simulink model "TRN"  (R2022a)
settings: Solver=FixedStepAuto  StartTime=0.0  StopTime=300  FixedStep=0.04  RelTol=1e-3
PreLoadFcn:
  | load('BusStructureTRNsensor.mat');
  | addpath('C:/MAP');
InitFcn:
  | %load TRNDataBusPILS.mat
  | %addpath(genpath(cd))
  | 
  | load('TPF_WHOLESIM_INPUT_SCENARIOS_AGCAS_N35_10E127_70.mat');
  | 
  | % Add DataBus Path
  | addpath(',,/');
  | addpath('../MAP/');
  | addpath('../MAP/MAP_DB');
  | addpath('../MAP/DVOF');
  | addpath(genpath(cd));
  | load('BusStructureTRN.mat');
undefined symbols (not defined in the file or in its folder): Altitude_INS, INSDataNotValid, Latitude_INS, Longitude_INS, TRN, TRNlib
libraries: simulink_extras x26, aerolibconvert2 x14, sharedtransform x3, dspstat3 x2
(part 2 of 3)

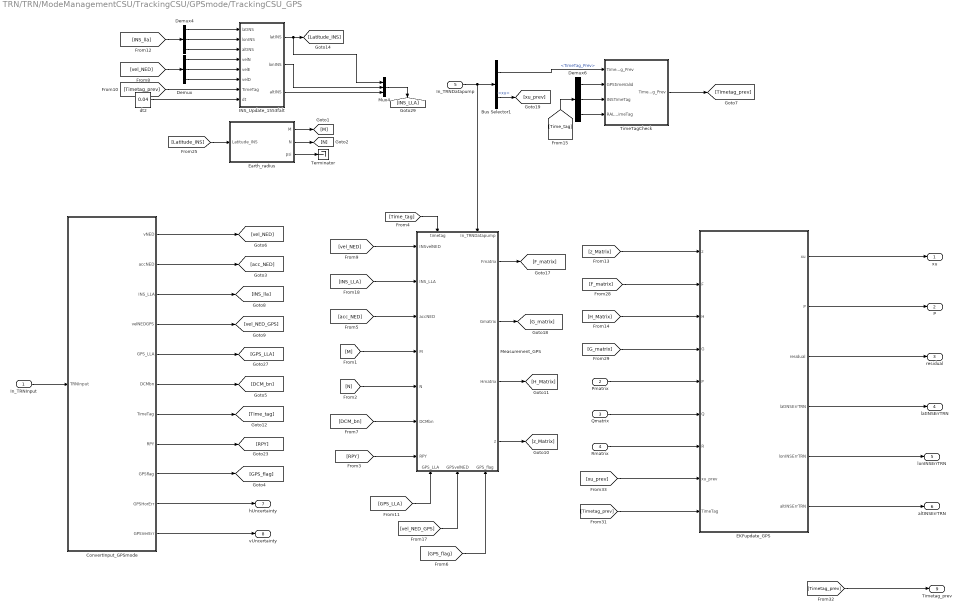
== system TRN/TRN/ModeManagementCSU/TrackingCSU/GPSmode/TrackingCSU_GPS ==
  In_TRNInput : Inport  OutDataTypeStr=Bus: TRNInput
  Pmatrix : Inport  Port=2
  Qmatrix : Inport  Port=3
  Rmatrix : Inport  Port=4
  In_TRNDatapump : Inport  Port=5  OutDataTypeStr=Bus: TRNDatapump  PortDimensions=1
  Bus Selector1 : BusSelector  OutputSignals=TimeTag_Prev,xu
  ConvertInput_GPSmode : Subsystem  TreatAsAtomicUnit=on
  Demux : Demux  Outputs=3
  Demux4 : Demux  Outputs=3
  Demux6 : Demux  Outputs=3
  EKFupdate_GPS : Subsystem
  Earth_radius : MATLAB Function  TreatAsAtomicUnit=on
  INS_Update_1553falt : MATLAB Function  TreatAsAtomicUnit=on
  Measurement_GPS : Subsystem
      settings: PortSchema="{\"entries\":[{\"content\":{\"sides\":[{\"content\":{\"connectorIds\":[\"In1\",\"In2\",\"In3\",\"In4\",\"In5\",\"In6\",\"In7\"]},\"type\":\"ConnectorPlacement.EquallySpacedRectSide\",\"uuid\":\"284c5e42-61c1-4616-966e-143f60f46571\"},{\"content\":{\"connectorIds\":[\"Out1\",\"Out2\",\"Out3\",\"Out4\"],\"side\":\"RIGHT\"},\"type\":\"ConnectorPlacement.EquallySpacedRectSide\",\"uuid\":\"be5b0b09-4e69-4cdf-8a94-a8639994cbf9\"},{\"content\":{\"connectorIds\":[\"In8\",\"In9\"],\"side\":\"TOP\"},\"type\":\"ConnectorPlacement.EquallySpacedRectSide\",\"uuid\":\"f7fbee8b-afe7-4fec-8c40-a5bd5e14374e\"},{\"content\":{\"connectorIds\":[\"In10\",\"In11\",\"In12\"],\"side\":\"BOTTOM\"},\"type\":\"ConnectorPlacement.EquallySpacedRectSide\",\"uuid\":\"9a503e43-aaca-441a-ab76-b52386228bc3\"}]},\"type\":\"ConnectorPlacement.EquallySpacedConnector\",\"uuid\":\"1b32203e-baad-4c49-8c24-20b6a9ecb4b9\"}],\"packageUris\":[\"http://schema.mathworks.com/mf0/Connector/R2020b\"],\"version\":\"1.0\"}"
  Mux4 : Mux  Inputs=3
  Terminator : Terminator
  TimeTagCheck : MATLAB Function  TreatAsAtomicUnit=on
  dt2 : Constant  Value=0.04  OutDataTypeStr=double
  xu : Outport
  P : Outport  Port=2
  residual : Outport  Port=3
  latINSErrTRN : Outport  Port=4
  lonINSErrTRN : Outport  Port=5
  altINSErrTRN : Outport  Port=6
  hUncertainty : Outport  Port=7
  vUncertainty : Outport  Port=8
  Timetag_prev : Outport  Port=9
  wires:
  Mux4/1 -> [INS_LLA]
  Demux/3 -> INS_Update_1553falt/6(velD)
  Demux/1 -> INS_Update_1553falt/4(velN)
  Demux/2 -> INS_Update_1553falt/5(velE)
  dt2/1 -> INS_Update_1553falt/8(dt)
  Bus Selector1/1 -> TimeTagCheck/1("TimeTag_Prev ")  "<TimeTag_Prev>"
  In_TRNDatapump/1 -> Bus Selector1/1, Measurement_GPS/9(In_TRNDatapump)
  INS_Update_1553falt/3(altINS) -> Mux4/3
  In_TRNInput/1 -> ConvertInput_GPSmode/1(TRNInput)
  INS_Update_1553falt/1(latINS) -> [Latitude_INS], Mux4/1
  INS_Update_1553falt/2(lonINS) -> Mux4/2
  ConvertInput_GPSmode/2(accNED) -> [acc_NED]
  ConvertInput_GPSmode/6(DCMbn) -> [DCM_bn]
  ConvertInput_GPSmode/1(vNED) -> [vel_NED]
  [vel_NED] -> Demux/1
  [Timetag_prev] -> INS_Update_1553falt/7(TimeTag)
  [INS_lla] -> Demux4/1
  Demux4/2 -> INS_Update_1553falt/2("lonINS ")
  Demux4/1 -> INS_Update_1553falt/1("latINS ")
  Demux4/3 -> INS_Update_1553falt/3("altINS ")
  ConvertInput_GPSmode/4(velNEDGPS) -> [vel_NED_GPS]
  [Time_tag] -> Demux6/1
  Demux6/1 -> TimeTagCheck/2(GPStimeValid)
  Demux6/2 -> TimeTagCheck/3(INSTimeTag)
  Demux6/3 -> TimeTagCheck/4(RALTTimeTag)
  [Timetag_prev] -> Timetag_prev/1
  Bus Selector1/2 -> [xu_prev]  "<xu>"
  Measurement_GPS/1(Fmatrix) -> [F_matrix]
  Measurement_GPS/2(Gmatrix) -> [G_matrix]
  Measurement_GPS/3(Hmatrix) -> [H_Matrix]
  Measurement_GPS/4(z) -> [z_Matrix]
  [z_Matrix] -> EKFupdate_GPS/1(z)
  [F_matrix] -> EKFupdate_GPS/2(F)
  [H_Matrix] -> EKFupdate_GPS/3(H)
  [G_matrix] -> EKFupdate_GPS/4(G)
  Pmatrix/1 -> EKFupdate_GPS/5("P ")
  Qmatrix/1 -> EKFupdate_GPS/6(Q)
  [xu_prev] -> EKFupdate_GPS/8(xu_prev)
  [Timetag_prev] -> EKFupdate_GPS/9(TimeTag)
  EKFupdate_GPS/1(xu) -> xu/1
  EKFupdate_GPS/2(P) -> P/1
  EKFupdate_GPS/3(residual) -> residual/1
  EKFupdate_GPS/4(latINSErrTRN) -> latINSErrTRN/1
  EKFupdate_GPS/5(lonINSErrTRN) -> lonINSErrTRN/1
  EKFupdate_GPS/6(altINSErrTRN) -> altINSErrTRN/1
  [vel_NED] -> Measurement_GPS/1(INSvelNED)
  [INS_LLA] -> Measurement_GPS/2(INS_LLA)
  [acc_NED] -> Measurement_GPS/3(accNED)
  [M] -> Measurement_GPS/4(M)
  [N] -> Measurement_GPS/5(N)
  [Latitude_INS] -> Earth_radius/1(Latitude_INS)
  Earth_radius/1(M) -> [M]
  Earth_radius/2(N) -> [N]
  ConvertInput_GPSmode/5(GPS_LLA) -> [GPS_LLA]
  [DCM_bn] -> Measurement_GPS/6(DCMbn)
  ConvertInput_GPSmode/8(RPY) -> [RPY]
  [RPY] -> Measurement_GPS/7(RPY)
  TimeTagCheck/1(TimeTag_Prev) -> [Timetag_prev]
  [GPS_LLA] -> Measurement_GPS/10(GPS_LLA)
  [vel_NED_GPS] -> Measurement_GPS/11(GPSvelNED)
  Rmatrix/1 -> EKFupdate_GPS/7(R)
  [Time_tag] -> Measurement_GPS/8(timetag)
  ConvertInput_GPSmode/9(GPSflag) -> [GPS_flag]
  [GPS_flag] -> Measurement_GPS/12(GPS_flag)
  ConvertInput_GPSmode/10(GPSHorErr) -> hUncertainty/1
  ConvertInput_GPSmode/11(GPSVerErr) -> vUncertainty/1
  ConvertInput_GPSmode/7(TimeTag) -> [Time_tag]
  ConvertInput_GPSmode/3(INS_LLA) -> [INS_lla]
  Earth_radius/3(psi) -> Terminator/1

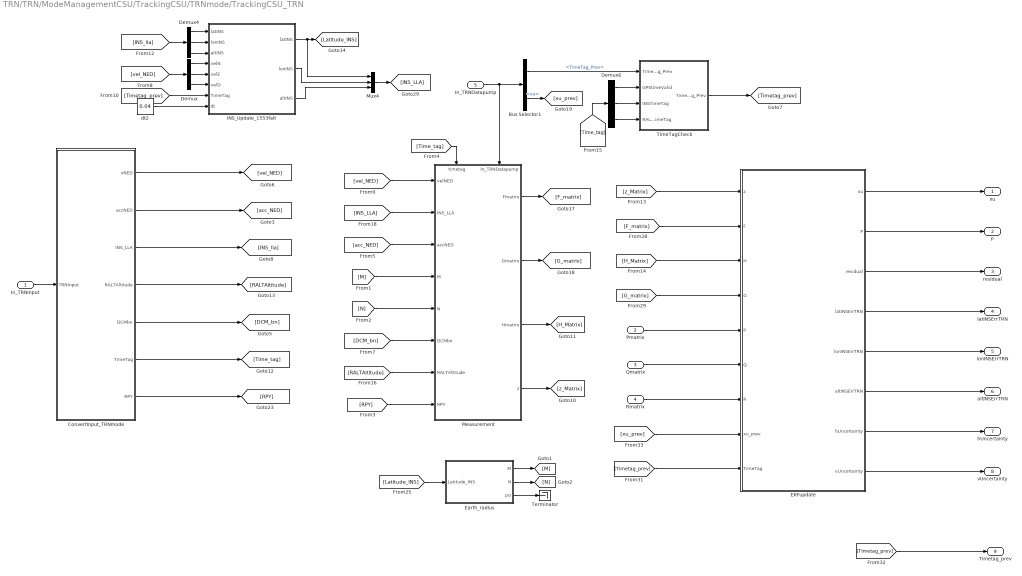
== system TRN/TRN/ModeManagementCSU/TrackingCSU/TRNmode/TrackingCSU_TRN ==
  In_TRNInput : Inport  OutDataTypeStr=Bus: TRNInput
  Pmatrix : Inport  Port=2
  Qmatrix : Inport  Port=3
  Rmatrix : Inport  Port=4
  In_TRNDatapump : Inport  Port=5  OutDataTypeStr=Bus: TRNDatapump  PortDimensions=1
  Bus Selector1 : BusSelector  OutputSignals=TimeTag_Prev,xu
  ConvertInput_TRNmode : Subsystem  TreatAsAtomicUnit=on
  Demux : Demux  Outputs=3
  Demux4 : Demux  Outputs=3
  Demux6 : Demux  Outputs=3
  EKFupdate : Subsystem
  Earth_radius : MATLAB Function  TreatAsAtomicUnit=on
  INS_Update_1553falt : MATLAB Function  TreatAsAtomicUnit=on
  Measurement : Subsystem
      settings: PortSchema="{\"entries\":[{\"content\":{\"sides\":[{\"content\":{\"connectorIds\":[\"In1\",\"In2\",\"In3\",\"In4\",\"In5\",\"In6\",\"In7\",\"In8\"]},\"type\":\"ConnectorPlacement.EquallySpacedRectSide\",\"uuid\":\"284c5e42-61c1-4616-966e-143f60f46571\"},{\"content\":{\"connectorIds\":[\"Out1\",\"Out2\",\"Out3\",\"Out4\"],\"side\":\"RIGHT\"},\"type\":\"ConnectorPlacement.EquallySpacedRectSide\",\"uuid\":\"be5b0b09-4e69-4cdf-8a94-a8639994cbf9\"},{\"content\":{\"connectorIds\":[\"In9\",\"In10\"],\"side\":\"TOP\"},\"type\":\"ConnectorPlacement.EquallySpacedRectSide\",\"uuid\":\"f7fbee8b-afe7-4fec-8c40-a5bd5e14374e\"}]},\"type\":\"ConnectorPlacement.EquallySpacedConnector\",\"uuid\":\"1b32203e-baad-4c49-8c24-20b6a9ecb4b9\"}],\"packageUris\":[\"http://schema.mathworks.com/mf0/Connector/R2020b\"],\"version\":\"1.0\"}"
  Mux4 : Mux  Inputs=3
  Terminator : Terminator
  TimeTagCheck : MATLAB Function  TreatAsAtomicUnit=on
  dt2 : Constant  Value=0.04  OutDataTypeStr=double
  xu : Outport
  P : Outport  Port=2
  residual : Outport  Port=3
  latINSErrTRN : Outport  Port=4
  lonINSErrTRN : Outport  Port=5
  altINSErrTRN : Outport  Port=6
  hUncertainty : Outport  Port=7
  vUncertainty : Outport  Port=8
  Timetag_prev : Outport  Port=9
  wires:
  TimeTagCheck/1(TimeTag_Prev) -> [Timetag_prev]
  [RPY] -> Measurement/8(RPY)
  ConvertInput_TRNmode/7(RPY) -> [RPY]
  [DCM_bn] -> Measurement/6(DCMbn)
  [RALTAltitude] -> Measurement/7(RALTAltitude)
  [N] -> Measurement/5(N)
  [M] -> Measurement/4(M)
  [acc_NED] -> Measurement/3(accNED)
  [INS_LLA] -> Measurement/2(INS_LLA)
  [vel_NED] -> Measurement/1(velNED)
  EKFupdate/7(hUncertainty) -> hUncertainty/1
  EKFupdate/6(altINSErrTRN) -> altINSErrTRN/1
  EKFupdate/5(lonINSErrTRN) -> lonINSErrTRN/1
  EKFupdate/4(latINSErrTRN) -> latINSErrTRN/1
  EKFupdate/8(vUncertainty) -> vUncertainty/1
  EKFupdate/3(residual) -> residual/1
  EKFupdate/2(P) -> P/1
  EKFupdate/1(xu) -> xu/1
  [Timetag_prev] -> EKFupdate/9(TimeTag)
  [xu_prev] -> EKFupdate/8(xu_prev)
  Rmatrix/1 -> EKFupdate/7(R)
  Qmatrix/1 -> EKFupdate/6(Q)
  Pmatrix/1 -> EKFupdate/5("P ")
  [G_matrix] -> EKFupdate/4(G)
  [H_Matrix] -> EKFupdate/3(H)
  [F_matrix] -> EKFupdate/2(F)
  [z_Matrix] -> EKFupdate/1(z)
  Measurement/4(z) -> [z_Matrix]
  Measurement/3(Hmatrix) -> [H_Matrix]
  Measurement/2(Gmatrix) -> [G_matrix]
  Measurement/1(Fmatrix) -> [F_matrix]
  Bus Selector1/2 -> [xu_prev]  "<xu>"
  [Timetag_prev] -> Timetag_prev/1
  ConvertInput_TRNmode/4(RALTAltitude) -> [RALTAltitude]
  Demux6/3 -> TimeTagCheck/4(RALTTimeTag)
  Demux6/2 -> TimeTagCheck/3(INSTimeTag)
  Demux6/1 -> TimeTagCheck/2(GPStimeValid)
  [Time_tag] -> Demux6/1
  Demux4/3 -> INS_Update_1553falt/3("altINS ")
  Demux4/1 -> INS_Update_1553falt/1("latINS ")
  Demux4/2 -> INS_Update_1553falt/2("lonINS ")
  [INS_lla] -> Demux4/1
  [Timetag_prev] -> INS_Update_1553falt/7(TimeTag)
  [vel_NED] -> Demux/1
  ConvertInput_TRNmode/1(vNED) -> [vel_NED]
  ConvertInput_TRNmode/5(DCMbn) -> [DCM_bn]
  ConvertInput_TRNmode/2(accNED) -> [acc_NED]
  INS_Update_1553falt/2(lonINS) -> Mux4/2
  INS_Update_1553falt/1(latINS) -> Mux4/1, [Latitude_INS]
  In_TRNInput/1 -> ConvertInput_TRNmode/1(TRNInput)
  INS_Update_1553falt/3(altINS) -> Mux4/3
  In_TRNDatapump/1 -> Measurement/10(In_TRNDatapump), Bus Selector1/1
  Bus Selector1/1 -> TimeTagCheck/1("TimeTag_Prev ")  "<TimeTag_Prev>"
  dt2/1 -> INS_Update_1553falt/8(dt)
  Demux/2 -> INS_Update_1553falt/5(velE)
  Demux/1 -> INS_Update_1553falt/4(velN)
  Demux/3 -> INS_Update_1553falt/6(velD)
  Mux4/1 -> [INS_LLA]
  [Time_tag] -> Measurement/9(timetag)
  ConvertInput_TRNmode/6(TimeTag) -> [Time_tag]
  ConvertInput_TRNmode/3(INS_LLA) -> [INS_lla]
  Earth_radius/2(N) -> [N]
  Earth_radius/1(M) -> [M]
  [Latitude_INS] -> Earth_radius/1(Latitude_INS)
  Earth_radius/3(psi) -> Terminator/1

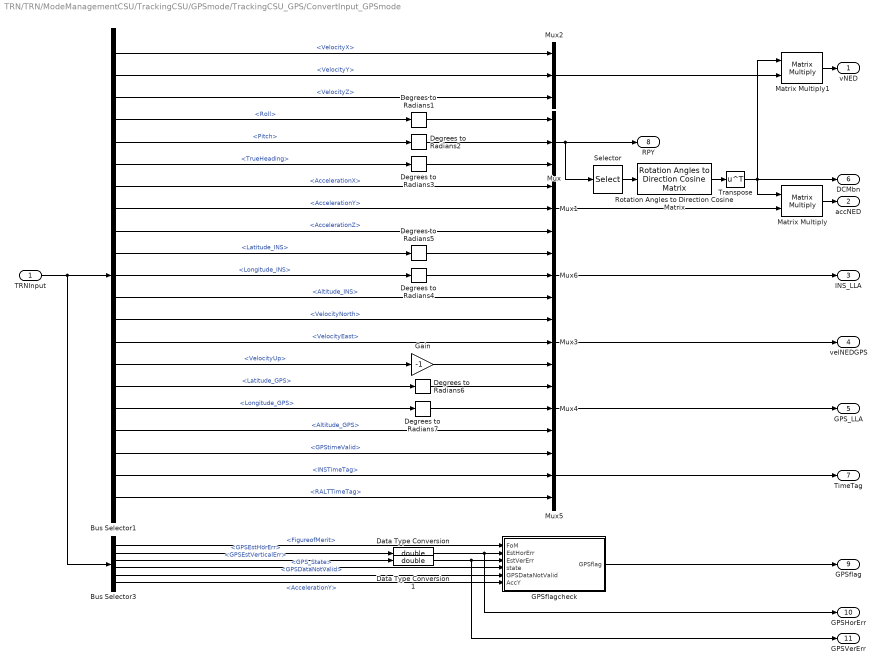
== system TRN/TRN/ModeManagementCSU/TrackingCSU/GPSmode/TrackingCSU_GPS/ConvertInput_GPSmode ==
  TRNInput : Inport
  Bus Selector1 : BusSelector  OutputSignals=VelocityX,VelocityY,VelocityZ,Roll,Pitch,TrueHeading,AccelerationX,AccelerationY,AccelerationZ,Latitude_INS,Longitude_INS,Altitude_INS,VelocityNorth,VelocityEast,VelocityUp,Latitude_GPS,Longitude_GPS,Altitude_GPS,GPStimeValid,INSTimeTag,RALTTimeTag
  Bus Selector3 : BusSelector  OutputSignals=FigureofMerit,GPSEstHorErr,GPSEstVerticalErr,GPS_State,GPSDataNotValid,AccelerationY
  Data Type Conversion : DataTypeConversion  OutDataTypeStr=double  SaturateOnIntegerOverflow=off  RndMeth=Floor
  Data Type Conversion1 : DataTypeConversion  OutDataTypeStr=double  SaturateOnIntegerOverflow=off  RndMeth=Floor
  Degrees to Radians{1..7} (7 alike) : simulink_extras/Transformations/Degrees to Radians
  GPSflagcheck : MATLAB Function  TreatAsAtomicUnit=on
  Gain : Gain  Gain=-1
  Matrix Multiply : Product  Multiplication=Matrix(*)
  Matrix Multiply1 : Product  Multiplication=Matrix(*)
  Mux{,1..6} (7 alike) : Mux  Inputs=3
  Rotation Angles to Direction Cosine Matrix : sharedtransform/Rotation Angles to Direction Cosine Matrix  rotationOrder=ZYX  aMode=aMode
      settings: SourceProductBaseCode=AE,PW,DR,MT,VE
  Selector : Selector  InputPortWidth=3  IndexOptions=Index vector (dialog)  Indices=[3 2 1]  OutputSizes=1
  Transpose : Math  Operator=transpose  SignedPower=on
  vNED : Outport  VectorParamsAs1DForOutWhenUnconnected=off
  accNED : Outport  Port=2  VectorParamsAs1DForOutWhenUnconnected=off
  INS_LLA : Outport  Port=3  VectorParamsAs1DForOutWhenUnconnected=off
  velNEDGPS : Outport  Port=4  VectorParamsAs1DForOutWhenUnconnected=off
  GPS_LLA : Outport  Port=5
  DCMbn : Outport  Port=6  VectorParamsAs1DForOutWhenUnconnected=off
  TimeTag : Outport  Port=7  VectorParamsAs1DForOutWhenUnconnected=off
  RPY : Outport  Port=8  VectorParamsAs1DForOutWhenUnconnected=off
  GPSflag : Outport  Port=9  VectorParamsAs1DForOutWhenUnconnected=off
  GPSHorErr : Outport  Port=10  VectorParamsAs1DForOutWhenUnconnected=off
  GPSVerErr : Outport  Port=11  VectorParamsAs1DForOutWhenUnconnected=off
  wires:
  Bus Selector1/18 -> Mux4/3  "<Altitude_GPS>"
  Bus Selector1/17 -> Degrees to Radians7/1  "<Longitude_GPS>"
  Degrees to Radians7/1 -> Mux4/2
  Bus Selector1/21 -> Mux5/3  "<RALTTimeTag>"
  Bus Selector1/20 -> Mux5/2  "<INSTimeTag>"
  Bus Selector1/19 -> Mux5/1  "<GPStimeValid>"
  Gain/1 -> Mux3/3
  Bus Selector1/15 -> Gain/1  "<VelocityUp>"
  Bus Selector1/14 -> Mux3/2  "<VelocityEast>"
  Bus Selector1/13 -> Mux3/1  "<VelocityNorth>"
  Bus Selector1/3 -> Mux2/3  "<VelocityZ>"
  Bus Selector1/1 -> Mux2/1  "<VelocityX>"
  Bus Selector1/4 -> Degrees to Radians1/1  "<Roll>"
  Bus Selector1/2 -> Mux2/2  "<VelocityY>"
  TRNInput/1 -> Bus Selector3/1, Bus Selector1/1
  Bus Selector1/6 -> Degrees to Radians3/1  "<TrueHeading>"
  Degrees to Radians2/1 -> Mux/2
  Degrees to Radians3/1 -> Mux/3
  Mux/1 -> Selector/1, RPY/1
  Bus Selector1/7 -> Mux1/1  "<AccelerationX>"
  Bus Selector1/5 -> Degrees to Radians2/1  "<Pitch>"
  Degrees to Radians1/1 -> Mux/1
  Bus Selector1/9 -> Mux1/3  "<AccelerationZ>"
  Bus Selector1/8 -> Mux1/2  "<AccelerationY>"
  Matrix Multiply1/1 -> vNED/1
  Matrix Multiply/1 -> accNED/1
  Mux1/1 -> Matrix Multiply/2
  Bus Selector1/10 -> Degrees to Radians5/1  "<Latitude_INS>"
  Transpose/1 -> Matrix Multiply/1, DCMbn/1, Matrix Multiply1/1
  Mux2/1 -> Matrix Multiply1/2
  Rotation Angles to Direction Cosine Matrix/1 -> Transpose/1
  Bus Selector1/11 -> Degrees to Radians4/1  "<Longitude_INS>"
  Degrees to Radians6/1 -> Mux4/1
  Bus Selector1/16 -> Degrees to Radians6/1  "<Latitude_GPS>"
  Selector/1 -> Rotation Angles to Direction Cosine Matrix/1
  Bus Selector3/2 -> Data Type Conversion/1  "<GPSEstHorErr>"
  Bus Selector3/1 -> GPSflagcheck/1(FoM)  "<FigureofMerit>"
  Bus Selector3/5 -> GPSflagcheck/5(GPSDataNotValid)  "<GPSDataNotValid>"
  Bus Selector3/3 -> Data Type Conversion1/1  "<GPSEstVerticalErr>"
  Bus Selector3/4 -> GPSflagcheck/4(state)  "<GPS_State>"
  Mux4/1 -> GPS_LLA/1
  Mux3/1 -> velNEDGPS/1
  GPSflagcheck/1(GPSflag) -> GPSflag/1
  Bus Selector3/6 -> GPSflagcheck/6(AccY)  "<AccelerationY>"
  Data Type Conversion/1 -> GPSHorErr/1, GPSflagcheck/2(EstHorErr)
  Data Type Conversion1/1 -> GPSVerErr/1, GPSflagcheck/3(EstVerErr)
  Mux5/1 -> TimeTag/1
  Degrees to Radians5/1 -> Mux6/1
  Degrees to Radians4/1 -> Mux6/2
  Bus Selector1/12 -> Mux6/3  "<Altitude_INS>"
  Mux6/1 -> INS_LLA/1

== system TRN/TRN/ModeManagementCSU/TrackingCSU/GPSmode/TrackingCSU_GPS/EKFupdate_GPS ==
  z : Inport
  F : Inport  Port=2
  H : Inport  Port=3
  G : Inport  Port=4
  "P " : Inport  Port=5
  Q : Inport  Port=6
  R : Inport  Port=7
  xu_prev : Inport  Port=8
  TimeTag : Inport  Port=9
  EKFUpdate_GPS : MATLAB Function  TreatAsAtomicUnit=on
  dt3 : Constant  Value=0.04  OutDataTypeStr=double
  xu : Outport
  P : Outport  Port=2
  residual : Outport  Port=3
  latINSErrTRN : Outport  Port=4
  lonINSErrTRN : Outport  Port=5
  altINSErrTRN : Outport  Port=6
  wires:
  R/1 -> EKFUpdate_GPS/7(R)
  H/1 -> EKFUpdate_GPS/3(H)
  "P "/1 -> EKFUpdate_GPS/5("P ")
  EKFUpdate_GPS/3(residual) -> residual/1
  TimeTag/1 -> EKFUpdate_GPS/10(TimeTag)
  F/1 -> EKFUpdate_GPS/2(F)
  xu_prev/1 -> EKFUpdate_GPS/9(xu_prev)
  G/1 -> EKFUpdate_GPS/4(G)
  EKFUpdate_GPS/1(xu) -> xu/1
  EKFUpdate_GPS/2(P) -> P/1
  Q/1 -> EKFUpdate_GPS/6(Q)
  z/1 -> EKFUpdate_GPS/1(z)
  dt3/1 -> EKFUpdate_GPS/8(dt)
  EKFUpdate_GPS/4(latINSErrTRN) -> latINSErrTRN/1
  EKFUpdate_GPS/5(lonINSErrTRN) -> lonINSErrTRN/1
  EKFUpdate_GPS/6(altINSErrTRN) -> altINSErrTRN/1

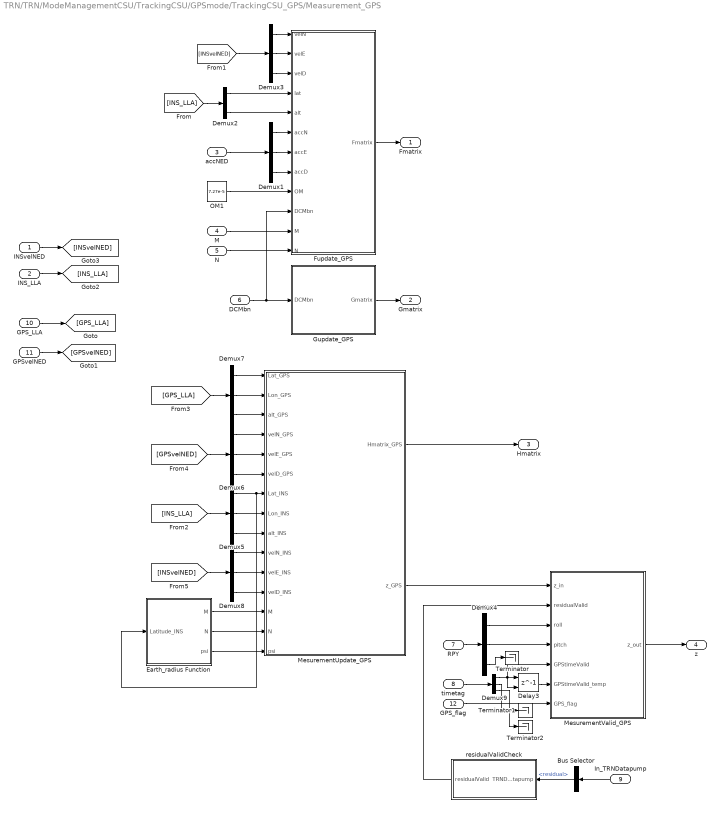
== system TRN/TRN/ModeManagementCSU/TrackingCSU/GPSmode/TrackingCSU_GPS/Measurement_GPS ==
  INSvelNED : Inport
  INS_LLA : Inport  Port=2
  accNED : Inport  Port=3
  M : Inport  Port=4
  N : Inport  Port=5
  DCMbn : Inport  Port=6
  RPY : Inport  Port=7
  timetag : Inport  Port=8
  In_TRNDatapump : Inport  Port=9
  GPS_LLA : Inport  Port=10
  GPSvelNED : Inport  Port=11
  GPS_flag : Inport  Port=12
  Bus Selector : BusSelector  OutputSignals=residual
  Delay3 : Delay  DelayLength=1  InitialConditionSource=Input port
      settings: InputPortMap=u0,p4
  Demux{1..9} (9 alike) : Demux  Outputs=3
  Earth_radius Function : MATLAB Function  TreatAsAtomicUnit=on
  Fupdate_GPS : MATLAB Function  TreatAsAtomicUnit=on
  Gupdate_GPS : MATLAB Function  TreatAsAtomicUnit=on
  MesurementUpdate_GPS : MATLAB Function  TreatAsAtomicUnit=on
  MesurementValid_GPS : MATLAB Function  TreatAsAtomicUnit=on
  OM1 : Constant  Value=7.27e-5
  Terminator : Terminator
  Terminator1 : Terminator
  Terminator2 : Terminator
  residualValidCheck : Subsystem
  Fmatrix : Outport
  Gmatrix : Outport  Port=2
  Hmatrix : Outport  Port=3
  z : Outport  Port=4
  wires:
  Demux1/3 -> Fupdate_GPS/8(accD)
  OM1/1 -> Fupdate_GPS/9(OM)
  Demux3/1 -> Fupdate_GPS/1(velN)
  Demux1/2 -> Fupdate_GPS/7(accE)
  Demux3/3 -> Fupdate_GPS/3(velD)
  Demux3/2 -> Fupdate_GPS/2(velE)
  Demux1/1 -> Fupdate_GPS/6(accN)
  Fupdate_GPS/1(Fmatrix) -> Fmatrix/1
  DCMbn/1 -> Gupdate_GPS/1(DCMbn), Fupdate_GPS/10(DCMbn)
  N/1 -> Fupdate_GPS/12(N)
  accNED/1 -> Demux1/1
  M/1 -> Fupdate_GPS/11(M)
  Demux2/1 -> Fupdate_GPS/4(lat)
  Demux2/3 -> Fupdate_GPS/5(alt)
  RPY/1 -> Demux4/1
  In_TRNDatapump/1 -> Bus Selector/1
  Bus Selector/1 -> residualValidCheck/1(TRNDatapump)  "<residual>"
  Demux5/1 -> Earth_radius Function/1(Latitude_INS), MesurementUpdate_GPS/7(Lat_INS)
  Demux5/2 -> MesurementUpdate_GPS/8(Lon_INS)
  Demux5/3 -> MesurementUpdate_GPS/9(alt_INS)
  Demux6/1 -> MesurementUpdate_GPS/4(velN_GPS)
  Demux6/2 -> MesurementUpdate_GPS/5(velE_GPS)
  Demux6/3 -> MesurementUpdate_GPS/6(velD_GPS)
  Demux7/1 -> MesurementUpdate_GPS/1(Lat_GPS)
  Demux7/2 -> MesurementUpdate_GPS/2(Lon_GPS)
  Demux7/3 -> MesurementUpdate_GPS/3(alt_GPS)
  Demux8/1 -> MesurementUpdate_GPS/10(velN_INS)
  Demux8/2 -> MesurementUpdate_GPS/11(velE_INS)
  Demux8/3 -> MesurementUpdate_GPS/12(velD_INS)
  Earth_radius Function/1(M) -> MesurementUpdate_GPS/13(M)
  Earth_radius Function/2(N) -> MesurementUpdate_GPS/14(N)
  Earth_radius Function/3(psi) -> MesurementUpdate_GPS/15(psi)
  GPS_LLA/1 -> [GPS_LLA]
  GPSvelNED/1 -> [GPSvelNED]
  INS_LLA/1 -> [INS_LLA]
  [INS_LLA] -> Demux2/1
  INSvelNED/1 -> [INSvelNED]
  [INSvelNED] -> Demux3/1
  [INS_LLA] -> Demux5/1
  [GPS_LLA] -> Demux7/1
  [GPSvelNED] -> Demux6/1
  [INSvelNED] -> Demux8/1
  MesurementUpdate_GPS/2(z_GPS) -> MesurementValid_GPS/1(z_in)
  MesurementUpdate_GPS/1(Hmatrix_GPS) -> Hmatrix/1
  Gupdate_GPS/1(Gmatrix) -> Gmatrix/1
  MesurementValid_GPS/1(z_out) -> z/1
  timetag/1 -> Demux9/1
  Delay3/1 -> MesurementValid_GPS/6(GPStimeValid_temp)
  Demux4/1 -> MesurementValid_GPS/3(roll)
  Demux4/2 -> MesurementValid_GPS/4(pitch)
  Demux9/1 -> Delay3/2, MesurementValid_GPS/5(GPStimeValid), Delay3/1
  residualValidCheck/1(residualValid) -> MesurementValid_GPS/2(residualValid)
  GPS_flag/1 -> MesurementValid_GPS/7(GPS_flag)
  Demux4/3 -> Terminator/1
  Demux9/2 -> Terminator1/1
  Demux9/3 -> Terminator2/1

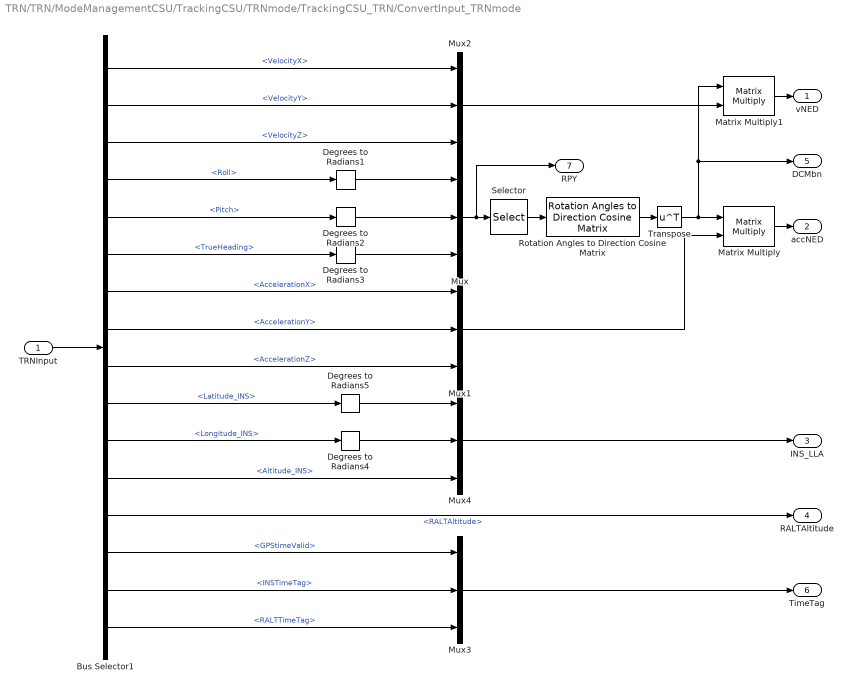
== system TRN/TRN/ModeManagementCSU/TrackingCSU/TRNmode/TrackingCSU_TRN/ConvertInput_TRNmode ==
  TRNInput : Inport
  Bus Selector1 : BusSelector  OutputSignals=VelocityX,VelocityY,VelocityZ,Roll,Pitch,TrueHeading,AccelerationX,AccelerationY,AccelerationZ,Latitude_INS,Longitude_INS,Altitude_INS,RALTAltitude,GPStimeValid,INSTimeTag,RALTTimeTag
  Degrees to Radians{1..5} (5 alike) : simulink_extras/Transformations/Degrees to Radians
  Matrix Multiply : Product  Multiplication=Matrix(*)
  Matrix Multiply1 : Product  Multiplication=Matrix(*)
  Mux{,1..4} (5 alike) : Mux  Inputs=3
  Rotation Angles to Direction Cosine Matrix : sharedtransform/Rotation Angles to Direction Cosine Matrix  rotationOrder=ZYX  aMode=aMode
      settings: SourceProductBaseCode=AE,PW,DR,MT,VE
  Selector : Selector  InputPortWidth=3  IndexOptions=Index vector (dialog)  Indices=[3 2 1]  OutputSizes=1
  Transpose : Math  Operator=transpose  SignedPower=on
  vNED : Outport  VectorParamsAs1DForOutWhenUnconnected=off
  accNED : Outport  Port=2  VectorParamsAs1DForOutWhenUnconnected=off
  INS_LLA : Outport  Port=3  VectorParamsAs1DForOutWhenUnconnected=off
  RALTAltitude : Outport  Port=4  VectorParamsAs1DForOutWhenUnconnected=off
  DCMbn : Outport  Port=5  VectorParamsAs1DForOutWhenUnconnected=off
  TimeTag : Outport  Port=6  VectorParamsAs1DForOutWhenUnconnected=off
  RPY : Outport  Port=7  VectorParamsAs1DForOutWhenUnconnected=off
  wires:
  Bus Selector1/11 -> Degrees to Radians4/1  "<Longitude_INS>"
  Rotation Angles to Direction Cosine Matrix/1 -> Transpose/1
  Mux2/1 -> Matrix Multiply1/2
  Transpose/1 -> Matrix Multiply/1, Matrix Multiply1/1, DCMbn/1
  Bus Selector1/10 -> Degrees to Radians5/1  "<Latitude_INS>"
  Mux1/1 -> Matrix Multiply/2
  Bus Selector1/13 -> RALTAltitude/1  "<RALTAltitude>"
  Matrix Multiply/1 -> accNED/1
  Matrix Multiply1/1 -> vNED/1
  Bus Selector1/8 -> Mux1/2  "<AccelerationY>"
  Bus Selector1/9 -> Mux1/3  "<AccelerationZ>"
  Degrees to Radians1/1 -> Mux/1
  Bus Selector1/5 -> Degrees to Radians2/1  "<Pitch>"
  Bus Selector1/7 -> Mux1/1  "<AccelerationX>"
  Mux/1 -> Selector/1, RPY/1
  Degrees to Radians3/1 -> Mux/3
  Degrees to Radians2/1 -> Mux/2
  Bus Selector1/6 -> Degrees to Radians3/1  "<TrueHeading>"
  TRNInput/1 -> Bus Selector1/1
  Bus Selector1/2 -> Mux2/2  "<VelocityY>"
  Bus Selector1/4 -> Degrees to Radians1/1  "<Roll>"
  Bus Selector1/1 -> Mux2/1  "<VelocityX>"
  Bus Selector1/3 -> Mux2/3  "<VelocityZ>"
  Selector/1 -> Rotation Angles to Direction Cosine Matrix/1
  Bus Selector1/14 -> Mux3/1  "<GPStimeValid>"
  Bus Selector1/15 -> Mux3/2  "<INSTimeTag>"
  Bus Selector1/16 -> Mux3/3  "<RALTTimeTag>"
  Mux3/1 -> TimeTag/1
  Degrees to Radians5/1 -> Mux4/1
  Degrees to Radians4/1 -> Mux4/2
  Bus Selector1/12 -> Mux4/3  "<Altitude_INS>"
  Mux4/1 -> INS_LLA/1

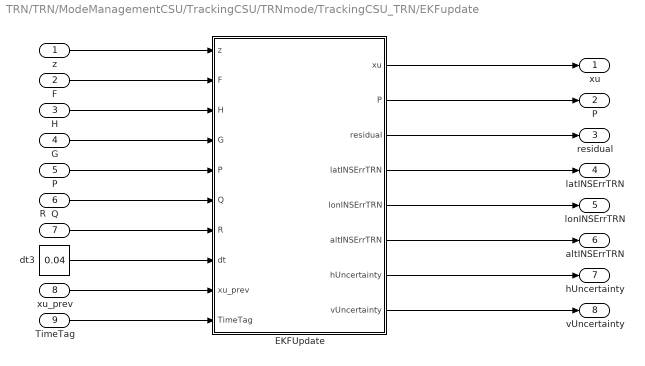
== system TRN/TRN/ModeManagementCSU/TrackingCSU/TRNmode/TrackingCSU_TRN/EKFupdate ==
  z : Inport
  F : Inport  Port=2
  H : Inport  Port=3
  G : Inport  Port=4
  "P " : Inport  Port=5
  Q : Inport  Port=6
  R : Inport  Port=7
  xu_prev : Inport  Port=8
  TimeTag : Inport  Port=9
  EKFUpdate : MATLAB Function  TreatAsAtomicUnit=on
  dt3 : Constant  Value=0.04  OutDataTypeStr=double
  xu : Outport
  P : Outport  Port=2
  residual : Outport  Port=3
  latINSErrTRN : Outport  Port=4
  lonINSErrTRN : Outport  Port=5
  altINSErrTRN : Outport  Port=6
  hUncertainty : Outport  Port=7
  vUncertainty : Outport  Port=8
  wires:
  EKFUpdate/7(hUncertainty) -> hUncertainty/1
  EKFUpdate/6(altINSErrTRN) -> altINSErrTRN/1
  EKFUpdate/5(lonINSErrTRN) -> lonINSErrTRN/1
  EKFUpdate/4(latINSErrTRN) -> latINSErrTRN/1
  dt3/1 -> EKFUpdate/8(dt)
  z/1 -> EKFUpdate/1(z)
  Q/1 -> EKFUpdate/6(Q)
  EKFUpdate/2(P) -> P/1
  EKFUpdate/1(xu) -> xu/1
  G/1 -> EKFUpdate/4(G)
  xu_prev/1 -> EKFUpdate/9(xu_prev)
  F/1 -> EKFUpdate/2(F)
  TimeTag/1 -> EKFUpdate/10(TimeTag)
  EKFUpdate/3(residual) -> residual/1
  EKFUpdate/8(vUncertainty) -> vUncertainty/1
  "P "/1 -> EKFUpdate/5("P ")
  H/1 -> EKFUpdate/3(H)
  R/1 -> EKFUpdate/7(R)

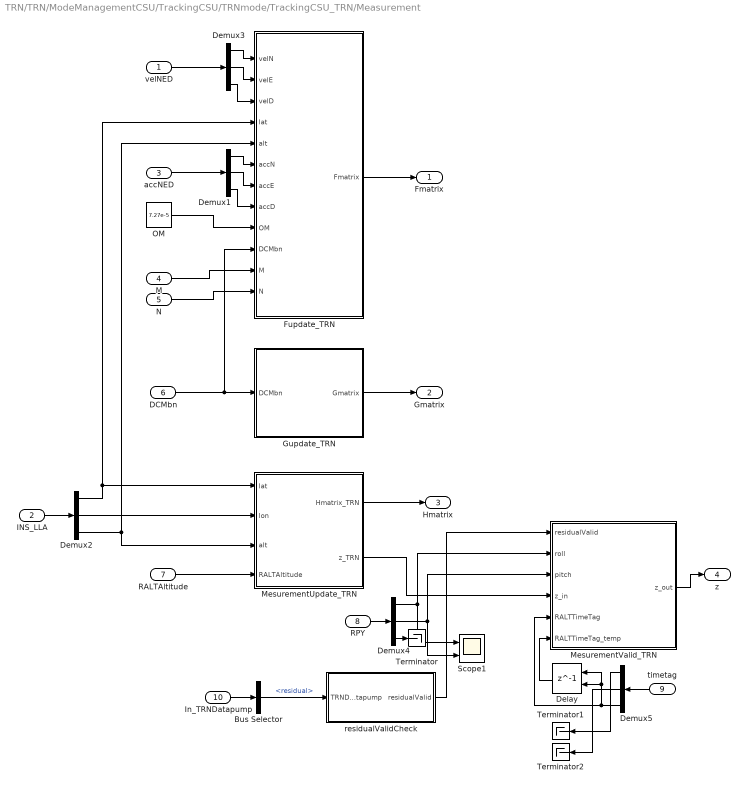
== system TRN/TRN/ModeManagementCSU/TrackingCSU/TRNmode/TrackingCSU_TRN/Measurement ==
  velNED : Inport
  INS_LLA : Inport  Port=2
  accNED : Inport  Port=3
  M : Inport  Port=4
  N : Inport  Port=5
  DCMbn : Inport  Port=6
  RALTAltitude : Inport  Port=7
  RPY : Inport  Port=8
  timetag : Inport  Port=9
  In_TRNDatapump : Inport  Port=10
  Bus Selector : BusSelector  OutputSignals=residual
  Delay : Delay  DelayLength=1  InitialConditionSource=Input port
      settings: InputPortMap=u0,p4
  Demux{1..5} (5 alike) : Demux  Outputs=3
  Fupdate_TRN : MATLAB Function  TreatAsAtomicUnit=on
  Gupdate_TRN : MATLAB Function  TreatAsAtomicUnit=on
  MesurementUpdate_TRN : MATLAB Function  TreatAsAtomicUnit=on
  MesurementValid_TRN : MATLAB Function  TreatAsAtomicUnit=on
  OM : Constant  Value=7.27e-5
  Scope1 : Scope  NumInputPorts=2
  Terminator : Terminator
  Terminator1 : Terminator
  Terminator2 : Terminator
  residualValidCheck : Subsystem
  Fmatrix : Outport
  Gmatrix : Outport  Port=2
  Hmatrix : Outport  Port=3
  z : Outport  Port=4
  wires:
  Bus Selector/1 -> residualValidCheck/1(TRNDatapump)  "<residual>"
  In_TRNDatapump/1 -> Bus Selector/1
  residualValidCheck/1(residualValid) -> MesurementValid_TRN/1(residualValid)
  MesurementValid_TRN/1(z_out) -> z/1
  Demux4/2 -> MesurementValid_TRN/3(pitch), Scope1/2
  Demux4/1 -> Scope1/1, MesurementValid_TRN/2(roll)
  RPY/1 -> Demux4/1
  Demux2/2 -> MesurementUpdate_TRN/2(lon)
  Demux2/3 -> Fupdate_TRN/5(alt), MesurementUpdate_TRN/3(alt)
  Demux2/1 -> MesurementUpdate_TRN/1(lat), Fupdate_TRN/4(lat)
  INS_LLA/1 -> Demux2/1
  MesurementUpdate_TRN/2(z_TRN) -> MesurementValid_TRN/4(z_in)
  MesurementUpdate_TRN/1(Hmatrix_TRN) -> Hmatrix/1
  M/1 -> Fupdate_TRN/11(M)
  velNED/1 -> Demux3/1
  accNED/1 -> Demux1/1
  N/1 -> Fupdate_TRN/12(N)
  DCMbn/1 -> Gupdate_TRN/1(DCMbn), Fupdate_TRN/10(DCMbn)
  Fupdate_TRN/1(Fmatrix) -> Fmatrix/1
  Gupdate_TRN/1(Gmatrix) -> Gmatrix/1
  Demux1/1 -> Fupdate_TRN/6(accN)
  Demux3/2 -> Fupdate_TRN/2(velE)
  Demux3/3 -> Fupdate_TRN/3(velD)
  RALTAltitude/1 -> MesurementUpdate_TRN/4(RALTAltitude)
  Demux1/2 -> Fupdate_TRN/7(accE)
  Demux3/1 -> Fupdate_TRN/1(velN)
  OM/1 -> Fupdate_TRN/9(OM)
  Demux1/3 -> Fupdate_TRN/8(accD)
  timetag/1 -> Demux5/1
  Demux5/3 -> MesurementValid_TRN/5(RALTTimeTag), Delay/1, Delay/2
  Delay/1 -> MesurementValid_TRN/6(RALTTimeTag_temp)
  Demux4/3 -> Terminator/1
  Demux5/1 -> Terminator1/1
  Demux5/2 -> Terminator2/1

== system TRN/TRN/ModeManagementCSU/TrackingCSU/GPSmode/TrackingCSU_GPS/Measurement_GPS/residualValidCheck ==
  TRNDatapump : Inport
  Bus Selector7 : BusSelector  OutputSignals=residual
  Data Type Conversion2 : DataTypeConversion  OutDataTypeStr=boolean  SaturateOnIntegerOverflow=off  RndMeth=Floor
  Gain2 : Gain  Gain=3
  Standard Deviation : dspstat3/Standard Deviation  run=on  directionMode=Entire input  dimension=1  reset_popup=None  roiEnable=off  roiType=Rectangles  roiPortion=Entire ROI  roiOutput=Individual statistics for each ROI  roiFlag=off
      settings: SourceProductBaseCode=DS
  Unit Delay3 : UnitDelay  SampleTime=-1  HasFrameUpgradeWarning=on
  residualCheck : MATLAB Function  TreatAsAtomicUnit=on
  residualValid : Outport
  wires:
  Bus Selector7/1 -> Standard Deviation/1, residualCheck/1(residual)  "<residual>"
  Unit Delay3/1 -> residualCheck/3("count ")
  TRNDatapump/1 -> Bus Selector7/1
  residualCheck/2(count) -> Unit Delay3/1
  Gain2/1 -> residualCheck/2(sigma_3)
  Standard Deviation/1 -> Gain2/1
  residualCheck/1(residualValid) -> Data Type Conversion2/1
  Data Type Conversion2/1 -> residualValid/1

== system TRN/TRN/ModeManagementCSU/TrackingCSU/TRNmode/TrackingCSU_TRN/Measurement/residualValidCheck ==
  TRNDatapump : Inport
  Bus Selector7 : BusSelector  OutputSignals=residual
  Data Type Conversion2 : DataTypeConversion  OutDataTypeStr=boolean  SaturateOnIntegerOverflow=off  RndMeth=Floor
  Gain2 : Gain  Gain=3
  Standard Deviation : dspstat3/Standard Deviation  run=on  directionMode=Entire input  dimension=1  reset_popup=None  roiEnable=off  roiType=Rectangles  roiPortion=Entire ROI  roiOutput=Individual statistics for each ROI  roiFlag=off
      settings: SourceProductBaseCode=DS
  Unit Delay3 : UnitDelay  SampleTime=-1  HasFrameUpgradeWarning=on
  residualCheck : MATLAB Function  TreatAsAtomicUnit=on
  residualValid : Outport
  wires:
  Bus Selector7/1 -> Standard Deviation/1, residualCheck/1(residual)  "<residual>"
  Unit Delay3/1 -> residualCheck/3("count ")
  TRNDatapump/1 -> Bus Selector7/1
  residualCheck/2(count) -> Unit Delay3/1
  Gain2/1 -> residualCheck/2(sigma_3)
  Standard Deviation/1 -> Gain2/1
  residualCheck/1(residualValid) -> Data Type Conversion2/1
  Data Type Conversion2/1 -> residualValid/1

== matlab function TRN/FlightPath_Angle/FlightPath_Angle ==
  data: vNED input; TRN_Ver_FlightPath_Angle output
function TRN_Ver_FlightPath_Angle  = FlightPath_Angle(vNED)

vN = vNED(1);
vE = vNED(2);
vD = vNED(3);

TRN_Ver_FlightPath_Angle = atan(-vD/sqrt(vN^2+vE^2));

== matlab function TRN/Terrain_0m_check ==
  data: Acq_hold output; hDEM input
function Acq_hold = Terrain_0m_check(hDEM)

persistent count
if(isempty(count))
    count = 0;
end

if (hDEM < 0.0000000001)
    count = count + 0.04;
else
    count = 0;
end

if count > 10
    Acq_hold = boolean(true);
else
    Acq_hold = boolean(false);
end

== stateflow chart TRN/ModeManagementCSU ==
  state Operation_In_Flight
    state Check_On_Terrain_Map [parallel]
      en, du:  Out_TRNOutput.AircraftOffTerrainMap = CheckOffTerrainMap(In_TRNInput.Latitude_INS, In_TRNInput.Longitude_INS);
      settings: executionOrder=1
    state Terrain_Referenced_Navigation [parallel]
      settings: executionOrder=2
      state On_Terrain_Map
        state Terrain_Map
          state TrackingCSU
            state ContinuousUpdate [parallel]
              en,du:  [xu,Pmatrix,residual,latINSErrTRN,lonINSErrTRN, ...
              altINSErrTRN,hUncertainty,vUncertainty, Out_TRNDatapump.TimeTag_Prev] = ...
              TrackingCSU(In_TRNInput,In_Pmatrix,Qmatrix, In_TRNDatapump);
              [continuousValid, Out_TRNOutput.NavigationMode]...
              = CheckValidity( hUncertainty, In_TRNInput.INSDataNotValid, Out_TRNDatapump.residual, In_TRNInput.INS_Alignment_State, ...
              In_TRNInput.GPSDataNotValid);
              settings: executionOrder=1
            state ValidityCheck [parallel]
              settings: executionOrder=2
              state ContinuousValid
                en, du:
                Out_TRNOutput.TRNEstOfINSLatitudeErr = latINSErrTRN * 180/pi;
                Out_TRNOutput.TRNEstOfINSLongitudeErr = lonINSErrTRN * 180/pi;
                Out_TRNOutput.TRNEstOfINSAltitudeErr = altINSErrTRN;
                Out_TRNOutput.AircraftPositionCorrectionValid = true;
              state ContinuousInValid
                en, du:
                Out_TRNOutput.TRNEstOfINSLatitudeErr = 0.0;
                Out_TRNOutput.TRNEstOfINSLongitudeErr = 0.0;
                Out_TRNOutput.TRNEstOfINSAltitudeErr = 0.0;
                Out_TRNOutput.AircraftPositionCorrectionValid = false;
              (default) -> ContinuousValid
              ContinuousValid -> ContinuousInValid : [continuousValid == false]
              ContinuousInValid -> ContinuousValid : [continuousValid == true]
            state UpdateContinuousParam_TRN [parallel]
              en, du:
              Out_TRNOutput.TRNHorUncertainty = hUncertainty * 6378000 * 25;
              Out_TRNOutput.TRNVerticalUncertainty = vUncertainty * 25;
              Out_TRNDatapump.xu = xu;
              Out_TRNDatapump.residual = residual;
              Out_Pmatrix = Pmatrix;
              settings: executionOrder=3
            state UpdateContinuousParam_GPS [parallel]
              en, du:
              Out_TRNOutput.TRNHorUncertainty = hUncertainty;
              Out_TRNOutput.TRNVerticalUncertainty = vUncertainty;
              Out_TRNDatapump.xu = xu;
              Out_TRNDatapump.residual = residual;
              Out_Pmatrix = Pmatrix;
              settings: executionOrder=4
            (default) -> (junction 407)
            (junction 407) -> UpdateContinuousParam_TRN [order 1] : [In_TRNInput.GPSDataNotValid == 1]
            (junction 407) -> UpdateContinuousParam_GPS [order 2] : [In_TRNInput.GPSDataNotValid == 0]
          state AcquisitionCSU
            state Batch_On
              state CollectProfile [parallel]
                en, du: [Out_TRNDatapump.MAD, Out_TRNDatapump.profileCnt, posUpdate, Out_TRNDatapump.residual] =...
                AcquisitionCSU(In_TRNInput,In_TRNDatapump)
                settings: executionOrder=1
              state CorrelationAnalysis [parallel]
                settings: executionOrder=2
                state BatchUpdate_On
                  en, du: Out_TRNOutput.TRNEstOfINSLatitudeErr = -posUpdate(1) * 180/pi;
                  Out_TRNOutput.TRNEstOfINSLongitudeErr = -posUpdate(2) * 180/pi;
                  Out_TRNDatapump.profileCnt = 0;
                  Out_TRNOutput.NavigationMode = false;
                  Out_TRNOutput.AircraftPositionCorrectionValid = true;
                  Out_Pmatrix = InitPmatrix();
                state BatchUpdate_Off
                  en, du: Out_TRNOutput.TRNEstOfINSLatitudeErr = 0.0;
                  Out_TRNOutput.TRNEstOfINSLongitudeErr = 0.0;
                  Out_TRNOutput.TRNEstOfINSAltitudeErr = 0.0;
                  Out_TRNOutput.NavigationMode = true;
                  Out_TRNOutput.AircraftPositionCorrectionValid = false;
                  Out_Pmatrix = InitPmatrix();
                (default) -> (junction 198)
                (junction 198) -> BatchUpdate_On [order 1] : [(Out_TRNDatapump.MAD <= 50&&...
                    | Out_TRNDatapump.profileCnt >= 20) || ...
                    |  (In_TRNInput.GPSDataNotValid == 0 && ...
                    | Out_TRNDatapump.MAD <= 50&&...
                    | Out_TRNDatapump.profileCnt >= 5)]
                (junction 198) -> BatchUpdate_Off [order 2]
            state Batch_Idle
              entry: Out_TRNOutput.TRNEstOfINSLatitudeErr = 0.0;
              Out_TRNOutput.TRNEstOfINSLongitudeErr = 0.0;
              Out_TRNOutput.NavigationMode = true;
              Out_TRNOutput.AircraftPositionCorrectionValid = false;
            (default) -> Batch_On
            Batch_Idle -> Batch_On : after(24, tick)
            Batch_On -> Batch_Idle : after(1, tick)
          (default) -> AcquisitionCSU
          TrackingCSU -> AcquisitionCSU : [In_TRNOutput.NavigationMode == true || ...
              | In_TRNInput.SoftResetRequest == true]
          AcquisitionCSU -> TrackingCSU : [In_TRNOutput.NavigationMode == false]
        state Terrain_height_Zero
          en, du:
          Out_TRNOutput.TRN_valid = true;
          Out_TRNOutput.TRNEstOfINSLatitudeErr = 0.0;
          Out_TRNOutput.TRNEstOfINSLongitudeErr = 0.0;
          Out_TRNOutput.TRNEstOfINSAltitudeErr = 0.0;
          Out_TRNOutput.NavigationMode = true;
          Out_TRNOutput.AircraftPositionCorrectionValid = false;
          Out_TRNDatapump.profileCnt = 0
        (default) -> Terrain_Map
        Terrain_Map -> Terrain_height_Zero : [In_TRNDatapump.Acq_hold == true && ...
            | In_TRNInput.GPSDataNotValid == 1]
        Terrain_height_Zero -> Terrain_Map : [In_TRNDatapump.Acq_hold == false]
      state Of_fTerrain_Map
      (default) -> On_Terrain_Map
      On_Terrain_Map -> Of_fTerrain_Map : [Out_TRNOutput.AircraftOffTerrainMap == true]
      Of_fTerrain_Map -> On_Terrain_Map : [Out_TRNOutput.AircraftOffTerrainMap == false]
  state Flight_Idle
    en, du:
    Out_TRNOutput.AircraftOffTerrainMap = CheckOffTerrainMap(In_TRNInput.Latitude_INS, In_TRNInput.Longitude_INS);
    Out_TRNOutput.TRN_valid = true;
    Out_TRNOutput.TRNEstOfINSLatitudeErr = 0.0;
    Out_TRNOutput.TRNEstOfINSLongitudeErr = 0.0;
    Out_TRNOutput.TRNEstOfINSAltitudeErr = 0.0;
    Out_TRNOutput.NavigationMode = false;
    Out_TRNOutput.AircraftPositionCorrectionValid = false;
  state [xu,Out_Pmatrix,residual,latINSErrTRN,lonINSErrTRN,altINSErrTRN,hUncertainty,vUncertainty,TimeTag_Prev] = TrackingCSU(In_TRNInput,In_Pmatrix,Qmatrix,In_TRNDatapump) [function]
  state [MAD,profileCnt,posUpdate,residual] = AcquisitionCSU(In_TRNInput,In_TRNDatapump) [function]
  (default) -> Operation_In_Flight
  Operation_In_Flight -> Flight_Idle : [In_TRNInput.WeightOnWheels == 1]
  Flight_Idle -> Operation_In_Flight : [In_TRNInput.WeightOnWheels == 0]
  data: In_TRNInput function_input Bus: TRNInput size=1 =0; In_Pmatrix function_input double size=[15 15]; Qmatrix function_input double size=[6 6]; xu function_output; Out_Pmatrix function_output; residual function_output; latINSErrTRN function_output; lonINSErrTRN function_output; altINSErrTRN function_output; hUncertainty function_output; vUncertainty function_output; In_TRNDatapump function_input Bus: TRNDatapump size=1; TimeTag_Prev function_output; In_TRNInput function_input Bus: TRNInput size=1 =0; In_TRNDatapump function_input Bus: TRNDatapump size=1 =0; MAD function_output; profileCnt function_output; posUpdate function_output; residual function_output; hUncertaintyTRN function_input; INSDataNotValid function_input; residualTRN function_input; valid function_output; navigationMode function_output; INS_Alignment_State function_input; GPSDataNotValid function_input; Pmat function_output double size=[15 15]; lat function_input; lon function_input; AircraftOffTerrainMap function_output; In_TRNInput input Bus: TRNInput; In_TRNOutput input Bus: TRNOutput; In_TRNDatapump input Bus: TRNDatapump; In_Pmatrix input double size=[15 15]; Out_TRNOutput output Bus: TRNOutput; Out_TRNDatapump output Bus: TRNDatapump; Qmatrix input double size=[6 6]; vUncertainty local double; lonINSErrTRN local double; latINSErrTRN local double; hUncertainty local double; altINSErrTRN local double; posUpdate local double; continuousValid local boolean; residual local double; xu local double size=15; Pmatrix local double size=[15 15]; Out_Pmatrix output double size=[15 15]
  function [valid, navigationMode] = CheckValidity(hUncertaintyTRN, INSDataNotValid, residualTRN, INS_Alignment_State, GPSDataNotValid):
    | function [valid, navigationMode] = CheckValidity(hUncertaintyTRN, INSDataNotValid, residualTRN, INS_Alignment_State, GPSDataNotValid)
    | 
    | persistent invalidCnt Count
    | if(isempty(invalidCnt))
    |     invalidCnt = 0;
    | end
    | if(isempty(Count))
    |     Count = 0;
    | end
    | 
    | if (residualTRN > 3 * std(residualTRN))
    |     Count = Count + 1;
    | else
    |     Count = 0;
    | 
    | end
    | 
    | if Count > 7
    |     weightedResidual = false;
    | else
    |     weightedResidual = true;
    | end
    | 
    | if GPSDataNotValid == 1
    |     % if(hUncertaintyTRN > (256))
    |     if(hUncertaintyTRN > (256 * 6378000 * 25)) || (INSDataNotValid == 1) || INS_Alignment_State == 0
    |         valid = false;
    |         invalidCnt = invalidCnt + 1;
    |     else
    |         valid = true;
    |         invalidCnt = 0;
    |     end
    | else
    |     if(hUncertaintyTRN > 256) || (INSDataNotValid == 1)
    |         valid = false;
    |         invalidCnt = invalidCnt + 1;
    |     else
    |         valid = true;
    |         invalidCnt = 0;
    |     end
    | end
    | 
    | if GPSDataNotValid == 1
    |     if (invalidCnt >= 50) || (INSDataNotValid == 1) || (weightedResidual == false)
    |     % if (invalidCnt >= 50) || (INSDataNotValid == 1)
    |         navigationMode = true;        % Acq CSU
    |     else
    |         navigationMode = false;       % Track CSU
    |     end
    | else
    |     if (invalidCnt >= 50)
    |         navigationMode = true;        % Acq CSU
    |     else
    |         navigationMode = false;       % Track CSU
    |     end
    | end
    | end
  function Pmat = InitPmatrix:
    | function Pmat = InitPmatrix()
    | 
    | R0      = 6378000;
    | 
    | attBias = [0 0 0];
    | velBias = [0 0 0];
    | posBias = [10 10 13.3] .* [1/R0 1/R0 1];
    | gyroBias = [0.4848e-6 0.4848e-6 0.4848e-6];
    | accBias = [2.9430e-4 2.9430e-4 2.9430e-4];
    | 
    | Pmat = diag([attBias velBias posBias gyroBias accBias].^2);
    | 
    | end
  function AircraftOffTerrainMap = CheckOffTerrainMap(lat, lon):
    | function AircraftOffTerrainMap = CheckOffTerrainMap(lat, lon)
    | 
    | AircraftTerrainMap = 0;
    | AircraftTerrainMap = coder.ceval('IsScanBoundary', lat, lon);     % InBoundary 1, NotBoundary 0
    | 
    | if(AircraftTerrainMap == 0)     % InBoundary 1, NotBoundary 0
    |     AircraftOffTerrainMap = true;
    | else
    |     AircraftOffTerrainMap = false;
    | end
    | 
    | end

== matlab function TRN/ModeManagementCSU/AcquisitionCSU/AcquisitionCSU/CorrelationAnalysis function ==
  data: batchProfile input; posUpdate output; profileCnt input; MAD output; resolution input; gridSize input; residual output; batchProfile output; lonTemp output; latTemp output; hDEM output; sum output
function [posUpdate, MAD, residual, batchProfile, lonTemp,latTemp,hDEM, sum] = CorrelationAnalysis(batchProfile, profileCnt, resolution, gridSize)
r2d = 180/pi;

posUpdate   = zeros(2,1);
MAD         = single(0);
sum         = 0;
latTemp     = 0;
lonTemp     = 0;
hDEM        = 0;
bestIdx     = [-999 -999];

gridRes  = 0.1;
MADTemp = 9999*ones(1,8000);

for i = -gridSize : gridSize
    for j = -gridSize : gridSize
        
        latTemp = batchProfile(((profileCnt-1)*(3+(gridSize+gridSize+1)*(gridSize+gridSize+1))) + 2) + i*gridRes*resolution;
        lonTemp = batchProfile(((profileCnt-1)*(3+(gridSize+gridSize+1)*(gridSize+gridSize+1))) + 3) + j*gridRes*resolution;
        hDEM    = coder.ceval('GetElevation', latTemp*r2d, lonTemp*r2d);

        batchProfile(((profileCnt-1)*(3+(gridSize+gridSize+1)*(gridSize+gridSize+1))) + 3 + ((i + gridSize) * (gridSize+gridSize+1)) + (j + gridSize + 1)) = abs(batchProfile(((profileCnt-1)*(3+(gridSize+gridSize+1)*(gridSize+gridSize+1))) + 1) - hDEM );   
    end
end

for i = 1 : (gridSize+gridSize+1) * (gridSize+gridSize+1)
    sum = 0;
    for j = 1 : profileCnt
        sum = sum + batchProfile(((j-1)*(3+(gridSize+gridSize+1)*(gridSize+gridSize+1))) + (i+3));
    end
    
    MADTemp(1,i) = sum/single(profileCnt);
    
end

[minMAD, minIdx] = min(MADTemp);
MAD = single(minMAD);
bestIdx(1) = floor(minIdx/(gridSize+gridSize+1));
bestIdx(2) = minIdx - (bestIdx(1) * (gridSize+gridSize+1));

if bestIdx(2) == 0
    bestIdx(1) = bestIdx(1) - 1;
    bestIdx(2) = (gridSize+gridSize);
end
%
bestIdx(1) = bestIdx(1) - gridSize;
bestIdx(2) = bestIdx(2) - gridSize - 1;
posUpdate(1) = bestIdx(1)*gridRes*resolution;
posUpdate(2) = bestIdx(2)*gridRes*resolution;

residual = double(MAD);

end

== matlab function TRN/ModeManagementCSU/AcquisitionCSU/AcquisitionCSU/StoreProfile function ==
  data: batchProfile input; batchProfile output; profileCnt input; latINS input; lonINS input; altINS input; RALT input; profileCnt output; gridSize output; latGPS input; lonGPS input; altGPS input; flagGPS input; flagINS input
function [batchProfile, profileCnt, gridSize] = StoreProfile(batchProfile, profileCnt, latINS, lonINS, altINS, RALT, latGPS, lonGPS, altGPS, flagGPS, flagINS)

gridSize = 20;

if(profileCnt >= 20)
      
    profileCnt = uint32(19);
    
    for i = 0:profileCnt-1
   
        for j = 1 : (3 + (gridSize + gridSize + 1) * (gridSize + gridSize + 1))
            batchProfile(i * (3 + (gridSize + gridSize + 1) * (gridSize + gridSize + 1)) + j) = batchProfile((i+1) * (3 + (gridSize + gridSize + 1) * (gridSize + gridSize + 1)) + j);
        end
    end
            
end

if flagGPS == 1
    batchProfile((profileCnt*(3+((gridSize + gridSize + 1) * (gridSize + gridSize + 1)))) + 1) = altINS - RALT;
    batchProfile((profileCnt*(3+((gridSize + gridSize + 1) * (gridSize + gridSize + 1)))) + 2) = latINS;
    batchProfile((profileCnt*(3+((gridSize + gridSize + 1) * (gridSize + gridSize + 1)))) + 3) = lonINS;
elseif flagGPS == 0
    batchProfile((profileCnt*(3+((gridSize + gridSize + 1) * (gridSize + gridSize + 1)))) + 1) = altGPS - RALT;
    batchProfile((profileCnt*(3+((gridSize + gridSize + 1) * (gridSize + gridSize + 1)))) + 2) = latGPS;
    batchProfile((profileCnt*(3+((gridSize + gridSize + 1) * (gridSize + gridSize + 1)))) + 3) = lonGPS;
end

if flagINS == 0
    profileCnt = profileCnt + 1;
elseif flagINS == 1
    profileCnt = uint32(0);
end

end

== matlab function TRN/ModeManagementCSU/TrackingCSU/GPSmode/TrackingCSU_GPS/ConvertInput_GPSmode/GPSflagcheck ==
  data: FoM input; GPSflag output; EstHorErr input; EstVerErr input; state input; GPSDataNotValid input; AccY input
function GPSflag  = GPScheck(FoM, EstHorErr, EstVerErr, state, GPSDataNotValid, AccY)
GPSflag = 2;
if GPSDataNotValid == 0
    if EstHorErr < 100 && EstVerErr < 25 && state == 5
        if FoM <= 4
            GPSflag = 1;
            if FoM <= 2 && AccY < 2
                GPSflag = 0;
            end
        end
    end
else
    GPSflag = 2;
end

== matlab function TRN/ModeManagementCSU/TrackingCSU/GPSmode/TrackingCSU_GPS/EKFupdate_GPS/EKFUpdate_GPS ==
  data: z input; xu output; P output; F input; H input; G input; P input; Q input; R input; dt input; residual output; latINSErrTRN output; lonINSErrTRN output; altINSErrTRN output; xu_prev input; TimeTag input
function [xu, P, residual, latINSErrTRN, lonINSErrTRN, altINSErrTRN] = EKFUpdate(z, F, H, G, P, Q, R, dt, xu_prev, TimeTag)

x = zeros(15,1);
I = eye(max(size(F)));

A = I + (F*dt);
Q = (A*G * Q * G'*A') .* dt;

%-------------------------------------%
% Predicts states & covariance matrix
%-------------------------------------%
xp = A * x;
Pp = (A * P * A') + Q;

%---------------------%
% Updates Kalman gain
%---------------------%
K = (Pp * H')/(R + H * Pp * H');

%----------------%
% Updates states
%----------------%
xu = xp + K * (z - H*xp);
% residual = z - H*xp;
residual = z(3);

%---------------------------%
% Updates covariance matrix
%---------------------------%
P = (I - K*H) * Pp * (I - K*H)' + K*R*K';


latINSErrTRN = xu(7);
lonINSErrTRN = xu(8);
altINSErrTRN = xu(9);

if TimeTag(4) == 1
    xu = xu_prev;
    latINSErrTRN = xu(7);
    lonINSErrTRN = xu(8);
    altINSErrTRN = xu(9);
end

end

== matlab function TRN/ModeManagementCSU/TrackingCSU/GPSmode/TrackingCSU_GPS/Earth_radius ==
  data: M output; N output; Latitude_INS input; psi output
function [M, N, psi] = Earth_radius(Latitude_INS)

    a   = 6378137;          % Earth's equatorial radius
    b   = 6356752.314245;   % Earth's polar radius
    psi = Latitude_INS;     % psi(latitude_INS)
    M   = ((a*b)^2) / ( ( (a*cos(psi))^2 + (b*sin(psi))^2 )^(3/2) );    % radius  of  curvature  in  meridian
    N   = (a^2) / ( ( (a*cos(psi))^2 + (b*sin(psi))^2 )^(1/2) );        % radius  of  curvature  in  prime  vertical

end

== matlab function TRN/DataProcess1/Subsystem3/Subsystem2/ConvertPlatformToBody ==
  data: vecPlatformXYZ input; vecBodyXYZ output; az_deg input
function vecBodyXYZ = ConvertPlatformToBody(vecPlatformXYZ, az_deg)
%CONVERTPLATFORMTOBODY

tformMat = diag([1, -1, -1]) * rotz( -az_deg );

vecBodyXYZ = tformMat * vecPlatformXYZ;

== matlab function TRN/ModeManagementCSU/TrackingCSU/GPSmode/TrackingCSU_GPS/INS_Update_1553falt ==
  data: latINS input; latINS output; lonINS input; altINS input; velN input; velE input; velD input; TimeTag input; lonINS output; altINS output; dt input
function [latINS, lonINS, altINS] = INS_Update_1553falt(latINS, lonINS, altINS, velN, velE, velD, TimeTag, dt)

R0 = 6378000;

if TimeTag(5) == 1
    latINS = latINS + (velN * dt) * 1/(R0+altINS);
    lonINS = lonINS + (velE * dt) * 1/(R0+altINS);
    altINS = altINS + (velD * dt) * 1/(R0+altINS);
end

== matlab function TRN/ModeManagementCSU/TrackingCSU/GPSmode/TrackingCSU_GPS/Measurement_GPS/Earth_radius Function ==
  data: M output; N output; psi output; Latitude_INS input
function [M, N, psi] = Earth_radius(Latitude_INS)

    a   = 6378137;          % Earth's equatorial radius
    b   = 6356752.314245;   % Earth's polar radius
    psi = Latitude_INS;     % psi(latitude_INS)
    M   = ((a*b)^2) / ( ( (a*cos(psi))^2 + (b*sin(psi))^2 )^(3/2) );    % radius  of  curvature  in  meridian
    N   = (a^2) / ( ( (a*cos(psi))^2 + (b*sin(psi))^2 )^(1/2) );        % radius  of  curvature  in  prime  vertical

end
